simulink model "uav_mission_supervisor"  (R2026a)
settings: Solver=FixedStepDiscrete  FixedStep=1.0
values from neighbouring files (symbols this model uses):
  Battery_Threshold_Critical = 10.0    [uav_mission_supervisor.sldd]
  Battery_Threshold_Low = 25.0    [uav_mission_supervisor.sldd]
settings Model: DataDictionary=uav_mission_supervisor.sldd  Creator=Nouran Ismail  LastModifiedBy=Nouran Ismail

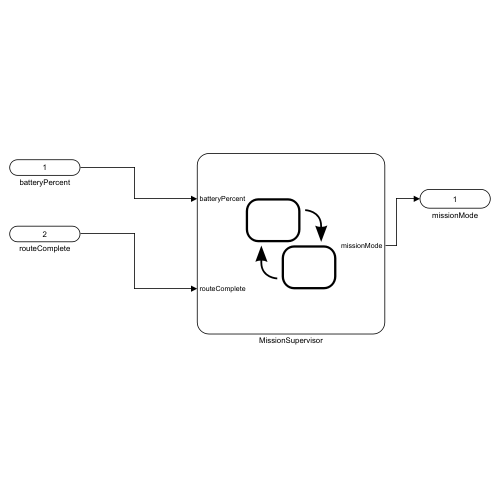
[thumbnail: Simulink's stored preview of the top-level diagram]
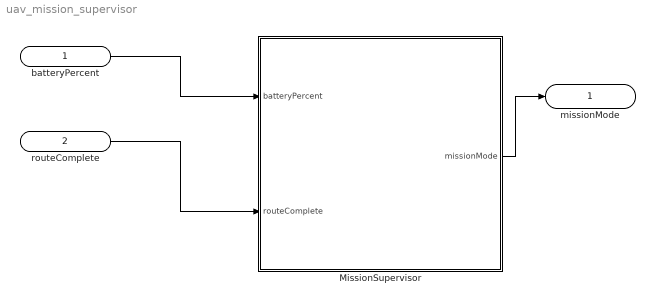
== system uav_mission_supervisor ==
  batteryPercent : Inport  OutMin=0  OutMax=100  OutDataTypeStr=double  Unit=percent  PortDimensions=1  SampleTime=1.0
  routeComplete : Inport  Port=2  OutDataTypeStr=boolean  Unit=1  PortDimensions=1  SampleTime=1.0
  MissionSupervisor : Stateflow chart  TreatAsAtomicUnit=on
  missionMode : Outport  OutDataTypeStr=Enum: MissionMode  Unit=1  PortDimensions=1
  wires:
  batteryPercent/1 -> MissionSupervisor/1(batteryPercent)
  routeComplete/1 -> MissionSupervisor/2(routeComplete)
  MissionSupervisor/1(missionMode) -> missionMode/1

== stateflow chart uav_mission_supervisor/MissionSupervisor ==
  state SafeLanding
    entry, during:
    missionMode = MissionMode.SafeLanding;
  state NormalInspection
    entry, during:
    missionMode = MissionMode.NormalInspection;
  state ReturnToHome
    entry, during:
    missionMode = MissionMode.ReturnToHome;
  state MissionComplete
    entry, during:
    missionMode = MissionMode.MissionComplete;
  (junction 17) -> SafeLanding [order 2] : [batteryPercent <= Battery_Threshold_Critical]
  NormalInspection -> SafeLanding [order 2] : [batteryPercent <= Battery_Threshold_Critical]
  NormalInspection -> SafeLanding [order 1] : [isnan(batteryPercent) || isinf(batteryPercent) || batteryPercent < 0 || batteryPercent > 100]
  (junction 17) -> SafeLanding [order 1] : [isnan(batteryPercent) || isinf(batteryPercent) || batteryPercent < 0 || batteryPercent > 100]
  ReturnToHome -> SafeLanding [order 2] : [batteryPercent <= Battery_Threshold_Critical]
  ReturnToHome -> SafeLanding [order 1] : [isnan(batteryPercent) || isinf(batteryPercent) || batteryPercent < 0 || batteryPercent > 100]
  (default) -> (junction 17)
  (junction 17) -> NormalInspection [order 5]
  (junction 17) -> ReturnToHome [order 3] : [batteryPercent <= Battery_Threshold_Low && batteryPercent > Battery_Threshold_Critical]
  (junction 17) -> MissionComplete [order 4] : [routeComplete == true]
  NormalInspection -> MissionComplete [order 4] : [routeComplete == true]
  NormalInspection -> ReturnToHome [order 3] : [batteryPercent <= Battery_Threshold_Low && batteryPercent > Battery_Threshold_Critical]
  data: batteryPercent input double; routeComplete input boolean; missionMode output Enum: MissionMode; Battery_Threshold_Low parameter double; Battery_Threshold_Critical parameter double
